simulink model "fdc_ut"  (Simulink 8.1)
settings: Solver=FixedStepDiscrete  StartTime=0.0  StopTime=Inf  FixedStep=0.005  RelTol=1e-3
libraries: siltestlib x6, fdc x1
settings Model: Creator=xsellart  LastModifiedBy=AT015555
settings DataIOCC: SignalLoggingSaveFormat=Dataset
settings OptimizationCC: ExpressionDepthLimit=128
settings DebuggingCC: FcnCallInpInsideContextMsg=EnableAllAsError
settings GRTTargetCC: CombineOutputUpdateFcns=on  GRTInterface=off

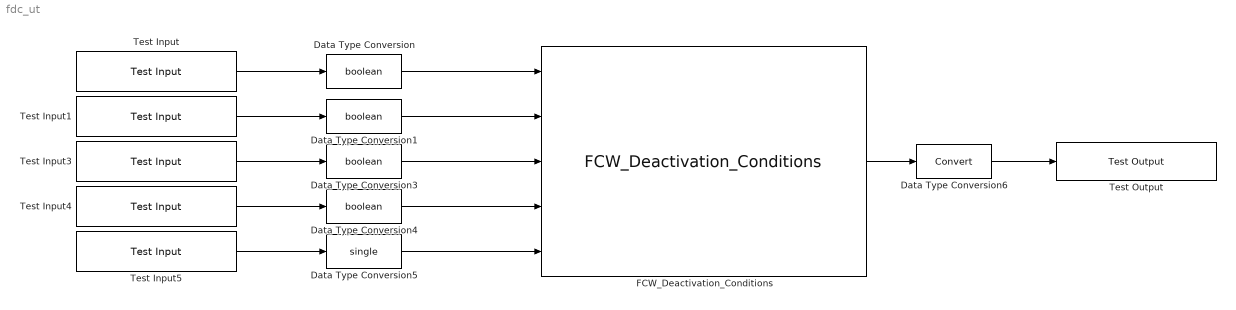
== system fdc_ut ==
  Data Type Conversion{,1,3..4} (4 alike) : DataTypeConversion  OutDataTypeStr=boolean
  Data Type Conversion5 : DataTypeConversion  OutDataTypeStr=single
  Data Type Conversion6 : DataTypeConversion
  FCW_Deactivation_Conditions : fdc/FCW_Deactivation_Conditions
  Test Input : siltestlib/Test Input  varname=VAEB_AEBActingPrev_flg  sampletime=0.005
  Test Input1 : siltestlib/Test Input  varname=VIFO_ParkingSituation_flg  sampletime=0.005
  Test Input3 : siltestlib/Test Input  varname=VIFO_DriverOverrideReq_flg  sampletime=0.005
  Test Input4 : siltestlib/Test Input  varname=VIFO_FCWTargetVehAssigned_flg  sampletime=0.005
  Test Input5 : siltestlib/Test Input  varname=VDINR_VehSpd_mps  sampletime=0.005
  Test Output : siltestlib/Test Output  varname=VJUD_FCWDeactivationReq_flg  sampletime=-1
  wires:
  Test Input/1 -> Data Type Conversion/1
  Data Type Conversion/1 -> FCW_Deactivation_Conditions/1
  Test Input1/1 -> Data Type Conversion1/1
  Data Type Conversion1/1 -> FCW_Deactivation_Conditions/2
  Test Input3/1 -> Data Type Conversion3/1
  Data Type Conversion4/1 -> FCW_Deactivation_Conditions/4
  Test Input4/1 -> Data Type Conversion4/1
  Data Type Conversion5/1 -> FCW_Deactivation_Conditions/5
  Test Input5/1 -> Data Type Conversion5/1
  FCW_Deactivation_Conditions/1 -> Data Type Conversion6/1
  Data Type Conversion6/1 -> Test Output/1
  Data Type Conversion3/1 -> FCW_Deactivation_Conditions/3
